simulink model "LUT_liver_pancreas_25"  (R2023b)
settings: Solver=FixedStepAuto  StartTime=0  StopTime=10.1  FixedStep=Timegap  RelTol=1e-3
model workspace (MAT data in the model file):
  T1_input = 1.34
(part 3 of 3)

== system LUT_liver_pancreas_25/If Action Subsystem6/If Action Subsystem2/If Action Subsystem9/If Action Subsystem1 ==
  In1 : Inport
  Action Port : ActionPort  ActionPortLabel=elseif( u1 >= 1.915)
  LUT 1.92RR : Lookup_n-D  NumberOfTableDimensions=1  BreakpointsForDimension1=[398.6604;505.5409;602.0864;698.3082;794.1288;889.6453;984.9397;1080.071;1175.08;1269.997;1364.843;1459.632;1554.377;1649.085;1743.765;1838.419;1933.054]  Table=[400;500;600;700;800;900;1000;1100;1200;1300;1400;1500;1600;1700;1800;1900;2000]  InternalRulePriority=Speed  RndMeth=Simplest
  Out1 : Outport
  wires:
  In1/1 -> LUT 1.92RR/1
  LUT 1.92RR/1 -> Out1/1

== system LUT_liver_pancreas_25/If Action Subsystem6/If Action Subsystem2/If Action Subsystem9/If Action Subsystem10 ==
  In1 : Inport
  Action Port : ActionPort  ActionPortLabel=if(u1 >= 1.995)
  LUT 2.00RR : Lookup_n-D  NumberOfTableDimensions=1  BreakpointsForDimension1=[398.4498;505.3086;601.8224;697.9817;793.713;889.1189;984.286;1079.277;1174.137;1268.896;1363.577;1458.198;1552.77;1647.302;1741.803;1836.277;1930.729]  Table=[400;500;600;700;800;900;1000;1100;1200;1300;1400;1500;1600;1700;1800;1900;2000]  InternalRulePriority=Speed  RndMeth=Simplest
  Out1 : Outport
  wires:
  In1/1 -> LUT 2.00RR/1
  LUT 2.00RR/1 -> Out1/1

== system LUT_liver_pancreas_25/If Action Subsystem6/If Action Subsystem2/If Action Subsystem9/If Action Subsystem11 ==
  In1 : Inport
  Action Port : ActionPort  ActionPortLabel=elseif( u1 >= 1.905)
  LUT 1.91RR : Lookup_n-D  NumberOfTableDimensions=1  BreakpointsForDimension1=[398.6878;505.5719;602.1224;698.3532;794.1862;889.7178;985.0294;1080.179;1175.209;1270.147;1365.014;1459.826;1554.593;1649.325;1744.028;1838.706;1933.365]  Table=[400;500;600;700;800;900;1000;1100;1200;1300;1400;1500;1600;1700;1800;1900;2000]  InternalRulePriority=Speed  RndMeth=Simplest
  Out1 : Outport
  wires:
  In1/1 -> LUT 1.91RR/1
  LUT 1.91RR/1 -> Out1/1

== system LUT_liver_pancreas_25/If Action Subsystem6/If Action Subsystem2/If Action Subsystem9/If Action Subsystem2 ==
  In1 : Inport
  Action Port : ActionPort  ActionPortLabel=else
  LUT 1.90RR : Lookup_n-D  NumberOfTableDimensions=1  BreakpointsForDimension1=[398.7156;505.6034;602.1591;698.3991;794.2449;889.7919;985.121;1080.29;1175.34;1270.299;1365.188;1460.023;1554.813;1649.569;1744.295;1838.998;1933.681]  Table=[400;500;600;700;800;900;1000;1100;1200;1300;1400;1500;1600;1700;1800;1900;2000]  InternalRulePriority=Speed  RndMeth=Simplest
  Out1 : Outport
  wires:
  In1/1 -> LUT 1.90RR/1
  LUT 1.90RR/1 -> Out1/1

== system LUT_liver_pancreas_25/If Action Subsystem6/If Action Subsystem2/If Action Subsystem9/If Action Subsystem3 ==
  In1 : Inport
  Action Port : ActionPort  ActionPortLabel=elseif( u1 >= 1.925)
  LUT 1.93RR : Lookup_n-D  NumberOfTableDimensions=1  BreakpointsForDimension1=[398.6331;505.5103;602.0511;698.2642;794.0727;889.5743;984.8519;1079.965;1174.954;1269.851;1364.675;1459.442;1554.164;1648.85;1743.505;1838.137;1932.747]  Table=[400;500;600;700;800;900;1000;1100;1200;1300;1400;1500;1600;1700;1800;1900;2000]  InternalRulePriority=Speed  RndMeth=Simplest
  Out1 : Outport
  wires:
  In1/1 -> LUT 1.93RR/1
  LUT 1.93RR/1 -> Out1/1

== system LUT_liver_pancreas_25/If Action Subsystem6/If Action Subsystem2/If Action Subsystem9/If Action Subsystem4 ==
  In1 : Inport
  Action Port : ActionPort  ActionPortLabel=elseif( u1 >= 1.935)
  LUT 1.94RR : Lookup_n-D  NumberOfTableDimensions=1  BreakpointsForDimension1=[398.6062;505.4802;602.0165;698.2211;794.0178;889.5049;984.7658;1079.86;1174.831;1269.706;1364.509;1459.255;1553.955;1648.618;1743.25;1837.858;1932.446]  Table=[400;500;600;700;800;900;1000;1100;1200;1300;1400;1500;1600;1700;1800;1900;2000]  InternalRulePriority=Speed  RndMeth=Simplest
  Out1 : Outport
  wires:
  In1/1 -> LUT 1.94RR/1
  LUT 1.94RR/1 -> Out1/1

== system LUT_liver_pancreas_25/If Action Subsystem6/If Action Subsystem2/If Action Subsystem9/If Action Subsystem5 ==
  In1 : Inport
  Action Port : ActionPort  ActionPortLabel=elseif( u1 >= 1.955)
  LUT 1.96RR : Lookup_n-D  NumberOfTableDimensions=1  BreakpointsForDimension1=[398.5531;505.4213;601.9493;698.1378;793.9116;889.3705;984.5991;1079.658;1174.59;1269.426;1364.187;1458.89;1553.546;1648.165;1742.752;1837.315;1931.856]  Table=[400;500;600;700;800;900;1000;1100;1200;1300;1400;1500;1600;1700;1800;1900;2000]  InternalRulePriority=Speed  RndMeth=Simplest
  Out1 : Outport
  wires:
  In1/1 -> LUT 1.96RR/1
  LUT 1.96RR/1 -> Out1/1

== system LUT_liver_pancreas_25/If Action Subsystem6/If Action Subsystem2/If Action Subsystem9/If Action Subsystem6 ==
  In1 : Inport
  Action Port : ActionPort  ActionPortLabel=elseif( u1 >= 1.945)
  LUT 1.95RR : Lookup_n-D  NumberOfTableDimensions=1  BreakpointsForDimension1=[398.5795;505.4506;601.9826;698.179;793.9641;889.437;984.6816;1079.758;1174.709;1269.565;1364.347;1459.071;1553.749;1648.389;1742.999;1837.585;1932.149]  Table=[400;500;600;700;800;900;1000;1100;1200;1300;1400;1500;1600;1700;1800;1900;2000]  InternalRulePriority=Speed  RndMeth=Simplest
  Out1 : Outport
  wires:
  In1/1 -> LUT 1.95RR/1
  LUT 1.95RR/1 -> Out1/1

== system LUT_liver_pancreas_25/If Action Subsystem6/If Action Subsystem2/If Action Subsystem9/If Action Subsystem7 ==
  In1 : Inport
  Action Port : ActionPort  ActionPortLabel=elseif( u1 >= 1.965)
  LUT 1.97RR : Lookup_n-D  NumberOfTableDimensions=1  BreakpointsForDimension1=[398.5269;505.3925;601.9166;698.0975;793.8603;889.3055;984.5183;1079.56;1174.473;1269.29;1364.031;1458.712;1553.347;1647.944;1742.509;1837.049;1931.568]  Table=[400;500;600;700;800;900;1000;1100;1200;1300;1400;1500;1600;1700;1800;1900;2000]  InternalRulePriority=Speed  RndMeth=Simplest
  Out1 : Outport
  wires:
  In1/1 -> LUT 1.97RR/1
  LUT 1.97RR/1 -> Out1/1

== system LUT_liver_pancreas_25/If Action Subsystem6/If Action Subsystem2/If Action Subsystem9/If Action Subsystem8 ==
  In1 : Inport
  Action Port : ActionPort  ActionPortLabel=elseif( u1 >= 1.975)
  LUT 1.98RR : Lookup_n-D  NumberOfTableDimensions=1  BreakpointsForDimension1=[398.501;505.3641;601.8846;698.058;793.8101;889.2419;984.4392;1079.464;1174.359;1269.156;1363.877;1458.538;1553.151;1647.726;1742.27;1836.788;1931.284]  Table=[400;500;600;700;800;900;1000;1100;1200;1300;1400;1500;1600;1700;1800;1900;2000]  InternalRulePriority=Speed  RndMeth=Simplest
  Out1 : Outport
  wires:
  In1/1 -> LUT 1.98RR/1
  LUT 1.98RR/1 -> Out1/1

== system LUT_liver_pancreas_25/If Action Subsystem6/If Action Subsystem2/If Action Subsystem9/If Action Subsystem9 ==
  In1 : Inport
  Action Port : ActionPort  ActionPortLabel=elseif(u1 >= 1.985)
  LUT 1.99RR : Lookup_n-D  NumberOfTableDimensions=1  BreakpointsForDimension1=[398.4753;505.3361;601.8532;698.0194;793.761;889.1797;984.3618;1079.369;1174.247;1269.025;1363.726;1458.366;1552.959;1647.513;1742.035;1836.53;1931.004]  Table=[400;500;600;700;800;900;1000;1100;1200;1300;1400;1500;1600;1700;1800;1900;2000]  InternalRulePriority=Speed  RndMeth=Simplest
  Out1 : Outport
  wires:
  In1/1 -> LUT 1.99RR/1
  LUT 1.99RR/1 -> Out1/1

== system LUT_liver_pancreas_25/If Action Subsystem6/If Action Subsystem3/If Action Subsystem5/If Action Subsystem1 ==
  In1 : Inport
  Action Port : ActionPort  ActionPortLabel=elseif( u1 >= 0.615)
  LUT 0.62RR : Lookup_n-D  NumberOfTableDimensions=1  BreakpointsForDimension1=[413.0526;530.6767;636.9684;743.5036;850.0094;956.4958;1063.005;1169.582;1276.273;1383.115;1490.11;1597.539;1705.059;1812.916;1921.116;2029.689;2138.661]  Table=[400;500;600;700;800;900;1000;1100;1200;1300;1400;1500;1600;1700;1800;1900;2000]  InternalRulePriority=Speed  RndMeth=Simplest
  Out1 : Outport
  wires:
  In1/1 -> LUT 0.62RR/1
  LUT 0.62RR/1 -> Out1/1

== system LUT_liver_pancreas_25/If Action Subsystem6/If Action Subsystem3/If Action Subsystem5/If Action Subsystem10 ==
  In1 : Inport
  Action Port : ActionPort  ActionPortLabel=elseif( u1 >= 0.605)
  LUT 0.61RR : Lookup_n-D  NumberOfTableDimensions=1  BreakpointsForDimension1=[413.6063;531.8654;638.6532;745.6537;852.6076;959.5359;1066.49;1173.523;1280.687;1388.021;1504.644;1603.565;1711.69;1820.197;1929.1;2038.429;2148.217]  Table=[400;500;600;700;800;900;1000;1100;1200;1300;1400;1500;1600;1700;1800;1900;2000]  InternalRulePriority=Speed  RndMeth=Simplest
  Out1 : Outport
  wires:
  In1/1 -> LUT 0.61RR/1
  LUT 0.61RR/1 -> Out1/1

== system LUT_liver_pancreas_25/If Action Subsystem6/If Action Subsystem3/If Action Subsystem5/If Action Subsystem2 ==
  In1 : Inport
  Action Port : ActionPort  ActionPortLabel=else
  LUT 0.6RR : Lookup_n-D  NumberOfTableDimensions=1  BreakpointsForDimension1=[414.1881;533.143;640.4713;747.9759;855.4138;962.8193;1070.254;1177.781;1285.457;1393.325;1505.695;1610.101;1718.894;1828.12;1937.801;2047.972;2158.67]  Table=[400;500;600;700;800;900;1000;1100;1200;1300;1400;1500;1600;1700;1800;1900;2000]  InternalRulePriority=Speed  RndMeth=Simplest
  Out1 : Outport
  wires:
  In1/1 -> LUT 0.6RR/1
  LUT 0.6RR/1 -> Out1/1

== system LUT_liver_pancreas_25/If Action Subsystem6/If Action Subsystem3/If Action Subsystem5/If Action Subsystem3 ==
  In1 : Inport
  Action Port : ActionPort  ActionPortLabel=elseif( u1 >= 0.625)
  LUT 0.63RR : Lookup_n-D  NumberOfTableDimensions=1  BreakpointsForDimension1=[412.5257;529.5692;635.4041;741.5087;847.5987;953.6745;1059.77;1165.926;1272.179;1378.566;1485.105;1591.969;1698.936;1806.202;1913.768;2021.658;2129.896]  Table=[400;500;600;700;800;900;1000;1100;1200;1300;1400;1500;1600;1700;1800;1900;2000]  InternalRulePriority=Speed  RndMeth=Simplest
  Out1 : Outport
  wires:
  In1/1 -> LUT 0.63RR/1
  LUT 0.63RR/1 -> Out1/1

== system LUT_liver_pancreas_25/If Action Subsystem6/If Action Subsystem3/If Action Subsystem5/If Action Subsystem4 ==
  In1 : Inport
  Action Port : ActionPort  ActionPortLabel=elseif( u1 >= 0.635)
  LUT 0.64RR : Lookup_n-D  NumberOfTableDimensions=1  BreakpointsForDimension1=[412.0245;528.5358;633.9491;739.6539;845.3569;951.0501;1056.761;1162.524;1268.371;1374.335;1480.441;1586.807;1693.265;1799.994;1906.983;2014.254;2121.83]  Table=[400;500;600;700;800;900;1000;1100;1200;1300;1400;1500;1600;1700;1800;1900;2000]  InternalRulePriority=Speed  RndMeth=Simplest
  Out1 : Outport
  wires:
  In1/1 -> LUT 0.64RR/1
  LUT 0.64RR/1 -> Out1/1

== system LUT_liver_pancreas_25/If Action Subsystem6/If Action Subsystem3/If Action Subsystem5/If Action Subsystem5 ==
  In1 : Inport
  Action Port : ActionPort  ActionPortLabel=elseif( u1 >= 0.655)
  LUT 0.66RR : Lookup_n-D  NumberOfTableDimensions=1  BreakpointsForDimension1=[411.0948;526.6663;631.3276;736.3133;841.3167;946.3174;1051.332;1156.386;1261.503;1366.708;1472.025;1580.011;1683.093;1788.878;1894.86;2001.057;2107.487]  Table=[400;500;600;700;800;900;1000;1100;1200;1300;1400;1500;1600;1700;1800;1900;2000]  InternalRulePriority=Speed  RndMeth=Simplest
  Out1 : Outport
  wires:
  In1/1 -> LUT 0.66RR/1
  LUT 0.66RR/1 -> Out1/1

== system LUT_liver_pancreas_25/If Action Subsystem6/If Action Subsystem3/If Action Subsystem5/If Action Subsystem6 ==
  In1 : Inport
  Action Port : ActionPort  ActionPortLabel=elseif( u1 >= 0.645)
  LUT 0.65RR : Lookup_n-D  NumberOfTableDimensions=1  BreakpointsForDimension1=[411.548;527.57;632.5933;737.9261;843.2677;948.6034;1053.955;1159.351;1264.821;1370.392;1476.091;1582.028;1687.998;1794.235;1900.698;2007.408;2114.383]  Table=[400;500;600;700;800;900;1000;1100;1200;1300;1400;1500;1600;1700;1800;1900;2000]  InternalRulePriority=Speed  RndMeth=Simplest
  Out1 : Outport
  wires:
  In1/1 -> LUT 0.65RR/1
  LUT 0.65RR/1 -> Out1/1

== system LUT_liver_pancreas_25/If Action Subsystem6/If Action Subsystem3/If Action Subsystem5/If Action Subsystem7 ==
  In1 : Inport
  Action Port : ActionPort  ActionPortLabel=elseif( u1 >= 0.665)
  LUT 0.67RR : Lookup_n-D  NumberOfTableDimensions=1  BreakpointsForDimension1=[410.6639;525.8193;630.1439;734.805;839.491;944.177;1048.876;1153.607;1258.394;1363.258;1468.219;1581.997;1678.512;1783.881;1889.421;1995.149;2101.08]  Table=[400;500;600;700;800;900;1000;1100;1200;1300;1400;1500;1600;1700;1800;1900;2000]  InternalRulePriority=Speed  RndMeth=Simplest
  Out1 : Outport
  wires:
  In1/1 -> LUT 0.67RR/1
  LUT 0.67RR/1 -> Out1/1

== system LUT_liver_pancreas_25/If Action Subsystem6/If Action Subsystem3/If Action Subsystem5/If Action Subsystem8 ==
  In1 : Inport
  Action Port : ActionPort  ActionPortLabel=elseif(u1 >= 0.675)
  LUT 0.68RR : Lookup_n-D  NumberOfTableDimensions=1  BreakpointsForDimension1=[410.2541;525.0244;629.0351;733.3917;837.7791;942.1686;1046.569;1150.998;1255.475;1360.018;1464.646;1569.375;1674.224;1779.207;1884.339;1989.636;2095.11]  Table=[400;500;600;700;800;900;1000;1100;1200;1300;1400;1500;1600;1700;1800;1900;2000]  InternalRulePriority=Speed  RndMeth=Simplest
  Out1 : Outport
  wires:
  In1/1 -> LUT 0.68RR/1
  LUT 0.68RR/1 -> Out1/1

== system LUT_liver_pancreas_25/If Action Subsystem6/If Action Subsystem3/If Action Subsystem5/If Action Subsystem9 ==
  In1 : Inport
  Action Port : ActionPort  ActionPortLabel=if(u1 >= 0.685)
  LUT 0.69RR : Lookup_n-D  NumberOfTableDimensions=1  BreakpointsForDimension1=[409.7732;524.2774;627.9946;732.0649;836.1708;940.2803;1044.4;1148.543;1252.728;1356.97;1461.285;1565.687;1670.201;1774.824;1879.579;1984.478;2089.532]  Table=[400;500;600;700;800;900;1000;1100;1200;1300;1400;1500;1600;1700;1800;1900;2000]  InternalRulePriority=Speed  RndMeth=Simplest
  Out1 : Outport
  wires:
  In1/1 -> LUT 0.69RR/1
  LUT 0.69RR/1 -> Out1/1

== system LUT_liver_pancreas_25/If Action Subsystem6/If Action Subsystem3/If Action Subsystem6/If Action Subsystem1 ==
  In1 : Inport
  Action Port : ActionPort  ActionPortLabel=elseif( u1 >= 0.515)
  LUT 0.52RR : Lookup_n-D  NumberOfTableDimensions=1  BreakpointsForDimension1=[419.925;547.8462;661.9676;775.6675;888.9962;1002.208;1115.536;1229.174;1343.225;1459.982;1574.478;1691.12;1808.984;1928.148;2048.731;2170.858;2294.661]  Table=[400;500;600;700;800;900;1000;1100;1200;1300;1400;1500;1600;1700;1800;1900;2000]  InternalRulePriority=Speed  RndMeth=Simplest
  Out1 : Outport
  wires:
  In1/1 -> LUT 0.52RR/1
  LUT 0.52RR/1 -> Out1/1

== system LUT_liver_pancreas_25/If Action Subsystem6/If Action Subsystem3/If Action Subsystem6/If Action Subsystem10 ==
  In1 : Inport
  Action Port : ActionPort  ActionPortLabel=elseif( u1 >= 0.505)
  LUT 0.51RR : Lookup_n-D  NumberOfTableDimensions=1  BreakpointsForDimension1=[420.7723;550.4608;665.9025;780.7905;895.2445;1009.57;1124.038;1238.87;1354.163;1471.848;1588.432;1706.804;1826.569;1947.837;2070.753;2195.464;2322.135]  Table=[400;500;600;700;800;900;1000;1100;1200;1300;1400;1500;1600;1700;1800;1900;2000]  InternalRulePriority=Speed  RndMeth=Simplest
  Out1 : Outport
  wires:
  In1/1 -> LUT 0.51RR/1
  LUT 0.51RR/1 -> Out1/1

== system LUT_liver_pancreas_25/If Action Subsystem6/If Action Subsystem3/If Action Subsystem6/If Action Subsystem2 ==
  In1 : Inport
  Action Port : ActionPort  ActionPortLabel=else
  LUT 0.50RR : Lookup_n-D  NumberOfTableDimensions=1  BreakpointsForDimension1=[421.6409;553.3122;670.2323;786.4478;902.1595;1017.731;1133.48;1249.661;1366.356;1485.421;1604.038;1724.383;1846.324;1970.008;2095.608;2223.304;2353.3]  Table=[400;500;600;700;800;900;1000;1100;1200;1300;1400;1500;1600;1700;1800;1900;2000]  InternalRulePriority=Speed  RndMeth=Simplest
  Out1 : Outport
  wires:
  In1/1 -> LUT 0.50RR/1
  LUT 0.50RR/1 -> Out1/1

== system LUT_liver_pancreas_25/If Action Subsystem6/If Action Subsystem3/If Action Subsystem6/If Action Subsystem3 ==
  In1 : Inport
  Action Port : ActionPort  ActionPortLabel=elseif( u1 >= 0.525)
  LUT 0.53RR : Lookup_n-D  NumberOfTableDimensions=1  BreakpointsForDimension1=[419.1032;545.4456;658.3845;771.0177;883.336;995.5501;1107.859;1220.432;1333.374;1450.068;1561.96;1677.078;1793.276;1910.599;2029.148;2149.026;2270.345]  Table=[400;500;600;700;800;900;1000;1100;1200;1300;1400;1500;1600;1700;1800;1900;2000]  InternalRulePriority=Speed  RndMeth=Simplest
  Out1 : Outport
  wires:
  In1/1 -> LUT 0.53RR/1
  LUT 0.53RR/1 -> Out1/1

== system LUT_liver_pancreas_25/If Action Subsystem6/If Action Subsystem3/If Action Subsystem6/If Action Subsystem4 ==
  In1 : Inport
  Action Port : ActionPort  ActionPortLabel=elseif( u1 >= 0.535)
  LUT 0.54RR : Lookup_n-D  NumberOfTableDimensions=1  BreakpointsForDimension1=[418.3095;543.2384;655.1154;766.7878;878.1954;989.5111;1100.905;1212.525;1324.473;1442.464;1550.696;1664.462;1779.194;1894.902;2011.67;2129.586;2248.743]  Table=[400;500;600;700;800;900;1000;1100;1200;1300;1400;1500;1600;1700;1800;1900;2000]  InternalRulePriority=Speed  RndMeth=Simplest
  Out1 : Outport
  wires:
  In1/1 -> LUT 0.54RR/1
  LUT 0.54RR/1 -> Out1/1

== system LUT_liver_pancreas_25/If Action Subsystem6/If Action Subsystem3/If Action Subsystem6/If Action Subsystem5 ==
  In1 : Inport
  Action Port : ActionPort  ActionPortLabel=elseif( u1 >= 0.555)
  LUT 0.56RR : Lookup_n-D  NumberOfTableDimensions=1  BreakpointsForDimension1=[416.8124;538.8983;649.3892;759.4066;869.2429;979.0103;1088.832;1198.821;1309.064;1419.513;1531.335;1642.805;1755.093;1868.119;1981.942;2096.624;2212.235]  Table=[400;500;600;700;800;900;1000;1100;1200;1300;1400;1500;1600;1700;1800;1900;2000]  InternalRulePriority=Speed  RndMeth=Simplest
  Out1 : Outport
  wires:
  In1/1 -> LUT 0.56RR/1
  LUT 0.56RR/1 -> Out1/1

== system LUT_liver_pancreas_25/If Action Subsystem6/If Action Subsystem3/If Action Subsystem6/If Action Subsystem6 ==
  In1 : Inport
  Action Port : ActionPort  ActionPortLabel=elseif( u1 >= 0.545)
  LUT 0.55RR : Lookup_n-D  NumberOfTableDimensions=1  BreakpointsForDimension1=[417.5456;541.1396;652.1268;762.9311;873.515;984.0188;1094.588;1205.35;1316.403;1436.98;1540.531;1653.091;1766.527;1880.812;1996.014;2112.21;2229.478]  Table=[400;500;600;700;800;900;1000;1100;1200;1300;1400;1500;1600;1700;1800;1900;2000]  InternalRulePriority=Speed  RndMeth=Simplest
  Out1 : Outport
  wires:
  In1/1 -> LUT 0.55RR/1
  LUT 0.55RR/1 -> Out1/1

== system LUT_liver_pancreas_25/If Action Subsystem6/If Action Subsystem3/If Action Subsystem6/If Action Subsystem7 ==
  In1 : Inport
  Action Port : ActionPort  ActionPortLabel=elseif( u1 >= 0.565)
  LUT 0.57RR : Lookup_n-D  NumberOfTableDimensions=1  BreakpointsForDimension1=[416.1104;536.8576;646.8766;756.1785;865.3339;974.4308;1083.574;1192.86;1302.37;1412.111;1523.01;1633.472;1744.736;1856.646;1969.247;2082.593;2196.744]  Table=[400;500;600;700;800;900;1000;1100;1200;1300;1400;1500;1600;1700;1800;1900;2000]  InternalRulePriority=Speed  RndMeth=Simplest
  Out1 : Outport
  wires:
  In1/1 -> LUT 0.57RR/1
  LUT 0.57RR/1 -> Out1/1

== system LUT_liver_pancreas_25/If Action Subsystem6/If Action Subsystem3/If Action Subsystem6/If Action Subsystem8 ==
  In1 : Inport
  Action Port : ActionPort  ActionPortLabel=elseif(u1 >= 0.575)
  LUT 0.58RR : Lookup_n-D  NumberOfTableDimensions=1  BreakpointsForDimension1=[415.4393;536.0008;644.566;753.2153;861.7484;970.2327;1078.756;1187.403;1296.246;1405.316;1515.517;1624.974;1735.325;1846.24;1957.755;2069.918;2182.779]  Table=[400;500;600;700;800;900;1000;1100;1200;1300;1400;1500;1600;1700;1800;1900;2000]  InternalRulePriority=Speed  RndMeth=Simplest
  Out1 : Outport
  wires:
  In1/1 -> LUT 0.58RR/1
  LUT 0.58RR/1 -> Out1/1

== system LUT_liver_pancreas_25/If Action Subsystem6/If Action Subsystem3/If Action Subsystem6/If Action Subsystem9 ==
  In1 : Inport
  Action Port : ActionPort  ActionPortLabel=if(u1 >= 0.585)
  LUT 0.59RR : Lookup_n-D  NumberOfTableDimensions=1  BreakpointsForDimension1=[414.7988;534.5182;642.4369;750.4892;858.4519;966.3743;1074.331;1182.393;1290.627;1399.073;1509.163;1617.212;1726.743;1836.769;1947.315;2058.426;2170.143]  Table=[400;500;600;700;800;900;1000;1100;1200;1300;1400;1500;1600;1700;1800;1900;2000]  InternalRulePriority=Speed  RndMeth=Simplest
  Out1 : Outport
  wires:
  In1/1 -> LUT 0.59RR/1
  LUT 0.59RR/1 -> Out1/1

== system LUT_liver_pancreas_25/If Action Subsystem6/If Action Subsystem3/If Action Subsystem7/If Action Subsystem1 ==
  In1 : Inport
  Action Port : ActionPort  ActionPortLabel=elseif( u1 >= 0.715)
  LUT 0.72RR : Lookup_n-D  NumberOfTableDimensions=1  BreakpointsForDimension1=[408.8044;522.2865;625.2275;728.5323;831.8808;935.2351;1038.595;1141.97;1245.37;1348.806;1452.289;1555.826;1661.357;1763.155;1866.924;1970.794;2074.77]  Table=[400;500;600;700;800;900;1000;1100;1200;1300;1400;1500;1600;1700;1800;1900;2000]  InternalRulePriority=Speed  RndMeth=Simplest
  Out1 : Outport
  wires:
  In1/1 -> LUT 0.72RR/1
  LUT 0.72RR/1 -> Out1/1

== system LUT_liver_pancreas_25/If Action Subsystem6/If Action Subsystem3/If Action Subsystem7/If Action Subsystem10 ==
  In1 : Inport
  Action Port : ActionPort  ActionPortLabel=elseif( u1 >= 0.705)
  LUT 0.71RR : Lookup_n-D  NumberOfTableDimensions=1  BreakpointsForDimension1=[409.1404;522.9118;626.0958;729.6417;833.2294;936.8226;1040.423;1144.041;1247.688;1351.378;1455.123;1558.931;1662.9;1766.82;1870.898;1975.087;2079.395]  Table=[400;500;600;700;800;900;1000;1100;1200;1300;1400;1500;1600;1700;1800;1900;2000]  InternalRulePriority=Speed  RndMeth=Simplest
  Out1 : Outport
  wires:
  In1/1 -> LUT 0.71RR/1
  LUT 0.71RR/1 -> Out1/1

== system LUT_liver_pancreas_25/If Action Subsystem6/If Action Subsystem3/If Action Subsystem7/If Action Subsystem2 ==
  In1 : Inport
  Action Port : ActionPort  ActionPortLabel=else
  LUT 0.70RR : Lookup_n-D  NumberOfTableDimensions=1  BreakpointsForDimension1=[409.5212;523.5744;627.0166;730.8172;834.657;938.5015;1042.354;1146.228;1250.137;1354.095;1458.116;1562.212;1666.423;1770.703;1875.108;1979.638;2084.306]  Table=[400;500;600;700;800;900;1000;1100;1200;1300;1400;1500;1600;1700;1800;1900;2000]  InternalRulePriority=Speed  RndMeth=Simplest
  Out1 : Outport
  wires:
  In1/1 -> LUT 0.70RR/1
  LUT 0.70RR/1 -> Out1/1

== system LUT_liver_pancreas_25/If Action Subsystem6/If Action Subsystem3/If Action Subsystem7/If Action Subsystem3 ==
  In1 : Inport
  Action Port : ActionPort  ActionPortLabel=elseif( u1 >= 0.725)
  LUT 0.73RR : Lookup_n-D  NumberOfTableDimensions=1  BreakpointsForDimension1=[408.4842;521.6957;624.4073;727.4836;830.6046;933.7314;1036.863;1140.006;1243.171;1346.366;1449.601;1552.882;1665.038;1759.687;1863.165;1966.738;2070.403]  Table=[400;500;600;700;800;900;1000;1100;1200;1300;1400;1500;1600;1700;1800;1900;2000]  InternalRulePriority=Speed  RndMeth=Simplest
  Out1 : Outport
  wires:
  In1/1 -> LUT 0.73RR/1
  LUT 0.73RR/1 -> Out1/1

== system LUT_liver_pancreas_25/If Action Subsystem6/If Action Subsystem3/If Action Subsystem7/If Action Subsystem4 ==
  In1 : Inport
  Action Port : ActionPort  ActionPortLabel=elseif( u1 >= 0.735)
  LUT 0.74RR : Lookup_n-D  NumberOfTableDimensions=1  BreakpointsForDimension1=[408.1791;521.1367;623.6316;726.4907;829.3949;932.3046;1035.218;1138.14;1241.08;1344.046;1447.047;1550.086;1653.132;1756.403;1859.603;1962.895;2066.27]  Table=[400;500;600;700;800;900;1000;1100;1200;1300;1400;1500;1600;1700;1800;1900;2000]  InternalRulePriority=Speed  RndMeth=Simplest
  Out1 : Outport
  wires:
  In1/1 -> LUT 0.74RR/1
  LUT 0.74RR/1 -> Out1/1

== system LUT_liver_pancreas_25/If Action Subsystem6/If Action Subsystem3/If Action Subsystem7/If Action Subsystem5 ==
  In1 : Inport
  Action Port : ActionPort  ActionPortLabel=elseif( u1 >= 0.755)
  LUT 0.76RR : Lookup_n-D  NumberOfTableDimensions=1  BreakpointsForDimension1=[407.6106;520.1046;622.1995;724.6547;827.1542;929.6577;1032.162;1134.671;1237.192;1339.732;1442.295;1544.886;1647.491;1750.366;1852.999;1955.777;2058.623]  Table=[400;500;600;700;800;900;1000;1100;1200;1300;1400;1500;1600;1700;1800;1900;2000]  InternalRulePriority=Speed  RndMeth=Simplest
  Out1 : Outport
  wires:
  In1/1 -> LUT 0.76RR/1
  LUT 0.76RR/1 -> Out1/1

== system LUT_liver_pancreas_25/If Action Subsystem6/If Action Subsystem3/If Action Subsystem7/If Action Subsystem6 ==
  In1 : Inport
  Action Port : ActionPort  ActionPortLabel=elseif( u1 >= 0.745)
  LUT 0.75RR : Lookup_n-D  NumberOfTableDimensions=1  BreakpointsForDimension1=[407.8882;520.607;622.8967;725.549;828.2464;930.9486;1033.653;1136.364;1239.09;1341.838;1444.614;1547.424;1650.246;1753.294;1856.219;1959.247;2062.35]  Table=[400;500;600;700;800;900;1000;1100;1200;1300;1400;1500;1600;1700;1800;1900;2000]  InternalRulePriority=Speed  RndMeth=Simplest
  Out1 : Outport
  wires:
  In1/1 -> LUT 0.75RR/1
  LUT 0.75RR/1 -> Out1/1

== system LUT_liver_pancreas_25/If Action Subsystem6/If Action Subsystem3/If Action Subsystem7/If Action Subsystem7 ==
  In1 : Inport
  Action Port : ActionPort  ActionPortLabel=elseif( u1 >= 0.765)
  LUT 0.77RR : Lookup_n-D  NumberOfTableDimensions=1  BreakpointsForDimension1=[407.3457;519.4328;621.5371;723.8041;826.1141;928.4272;1030.74;1133.055;1235.38;1337.719;1440.079;1542.462;1644.858;1747.712;1849.931;1952.47;2055.074]  Table=[400;500;600;700;800;900;1000;1100;1200;1300;1400;1500;1600;1700;1800;1900;2000]  InternalRulePriority=Speed  RndMeth=Simplest
  Out1 : Outport
  wires:
  In1/1 -> LUT 0.77RR/1
  LUT 0.77RR/1 -> Out1/1

== system LUT_liver_pancreas_25/If Action Subsystem6/If Action Subsystem3/If Action Subsystem7/If Action Subsystem8 ==
  In1 : Inport
  Action Port : ActionPort  ActionPortLabel=elseif(u1 >= 0.775)
  LUT 0.78RR : Lookup_n-D  NumberOfTableDimensions=1  BreakpointsForDimension1=[407.0925;519.1024;620.9069;722.9938;825.1221;927.2523;1029.38;1131.51;1233.646;1335.794;1437.959;1540.144;1642.339;1746.985;1847.004;1949.313;2051.688]  Table=[400;500;600;700;800;900;1000;1100;1200;1300;1400;1500;1600;1700;1800;1900;2000]  InternalRulePriority=Speed  RndMeth=Simplest
  Out1 : Outport
  wires:
  In1/1 -> LUT 0.78RR/1
  LUT 0.78RR/1 -> Out1/1

== system LUT_liver_pancreas_25/If Action Subsystem6/If Action Subsystem3/If Action Subsystem7/If Action Subsystem9 ==
  In1 : Inport
  Action Port : ActionPort  ActionPortLabel=if(u1 >= 0.785)
  LUT 0.79RR : Lookup_n-D  NumberOfTableDimensions=1  BreakpointsForDimension1=[406.8506;518.7905;620.3067;722.221;824.1748;926.1291;1028.08;1130.03;1231.986;1333.95;1435.928;1537.922;1639.926;1741.712;1844.209;1946.294;2048.451]  Table=[400;500;600;700;800;900;1000;1100;1200;1300;1400;1500;1600;1700;1800;1900;2000]  InternalRulePriority=Speed  RndMeth=Simplest
  Out1 : Outport
  wires:
  In1/1 -> LUT 0.79RR/1
  LUT 0.79RR/1 -> Out1/1

== system LUT_liver_pancreas_25/If Action Subsystem6/If Action Subsystem3/If Action Subsystem8/If Action Subsystem1 ==
  In1 : Inport
  Action Port : ActionPort  ActionPortLabel=elseif( u1 >= 0.815)
  LUT 0.82RR : Lookup_n-D  NumberOfTableDimensions=1  BreakpointsForDimension1=[406.1853;517.5611;618.6645;720.1013;821.5701;923.0343;1024.491;1125.942;1227.393;1328.846;1430.306;1531.774;1633.247;1734.683;1836.627;1937.969;2039.525]  Table=[400;500;600;700;800;900;1000;1100;1200;1300;1400;1500;1600;1700;1800;1900;2000]  InternalRulePriority=Speed  RndMeth=Simplest
  Out1 : Outport
  wires:
  In1/1 -> LUT 0.82RR/1
  LUT 0.82RR/1 -> Out1/1

== system LUT_liver_pancreas_25/If Action Subsystem6/If Action Subsystem3/If Action Subsystem8/If Action Subsystem10 ==
  In1 : Inport
  Action Port : ActionPort  ActionPortLabel=elseif( u1 >= 0.805)
  LUT 0.81RR : Lookup_n-D  NumberOfTableDimensions=1  BreakpointsForDimension1=[406.3976;517.9366;619.1873;720.7771;822.4016;924.0233;1025.639;1127.251;1228.863;1330.481;1432.107;1533.744;1635.387;1736.972;1839.006;1940.63;2042.379]  Table=[400;500;600;700;800;900;1000;1100;1200;1300;1400;1500;1600;1700;1800;1900;2000]  InternalRulePriority=Speed  RndMeth=Simplest
  Out1 : Outport
  wires:
  In1/1 -> LUT 0.81RR/1
  LUT 0.81RR/1 -> Out1/1

== system LUT_liver_pancreas_25/If Action Subsystem6/If Action Subsystem3/If Action Subsystem8/If Action Subsystem2 ==
  In1 : Inport
  Action Port : ActionPort  ActionPortLabel=else
  LUT 0.80RR : Lookup_n-D  NumberOfTableDimensions=1  BreakpointsForDimension1=[406.6191;518.4954;619.7341;721.4829;823.2689;925.0539;1026.834;1128.612;1230.393;1332.181;1433.979;1535.791;1637.611;1739.331;1841.542;1943.403;2045.351]  Table=[400;500;600;700;800;900;1000;1100;1200;1300;1400;1500;1600;1700;1800;1900;2000]  InternalRulePriority=Speed  RndMeth=Simplest
  Out1 : Outport
  wires:
  In1/1 -> LUT 0.80RR/1
  LUT 0.80RR/1 -> Out1/1

== system LUT_liver_pancreas_25/If Action Subsystem6/If Action Subsystem3/If Action Subsystem8/If Action Subsystem3 ==
  In1 : Inport
  Action Port : ActionPort  ActionPortLabel=elseif( u1 >= 0.825)
  LUT 0.83RR : Lookup_n-D  NumberOfTableDimensions=1  BreakpointsForDimension1=[405.9819;517.202;618.1641;719.4536;820.7721;922.0842;1023.387;1124.683;1225.977;1327.272;1428.572;1529.877;1631.187;1732.47;1834.573;1935.412;2036.78]  Table=[400;500;600;700;800;900;1000;1100;1200;1300;1400;1500;1600;1700;1800;1900;2000]  InternalRulePriority=Speed  RndMeth=Simplest
  Out1 : Outport
  wires:
  In1/1 -> LUT 0.83RR/1
  LUT 0.83RR/1 -> Out1/1

== system LUT_liver_pancreas_25/If Action Subsystem6/If Action Subsystem3/If Action Subsystem8/If Action Subsystem4 ==
  In1 : Inport
  Action Port : ActionPort  ActionPortLabel=elseif( u1 >= 0.835)
  LUT 0.84RR : Lookup_n-D  NumberOfTableDimensions=1  BreakpointsForDimension1=[405.7867;516.8582;617.6845;718.8321;820.0055;921.1704;1022.324;1123.471;1224.613;1325.755;1426.9;1528.049;1629.2;1730.332;1834.661;1932.955;2034.138]  Table=[400;500;600;700;800;900;1000;1100;1200;1300;1400;1500;1600;1700;1800;1900;2000]  InternalRulePriority=Speed  RndMeth=Simplest
  Out1 : Outport
  wires:
  In1/1 -> LUT 0.84RR/1
  LUT 0.84RR/1 -> Out1/1

== system LUT_liver_pancreas_25/If Action Subsystem6/If Action Subsystem3/If Action Subsystem8/If Action Subsystem5 ==
  In1 : Inport
  Action Port : ActionPort  ActionPortLabel=elseif( u1 >= 0.855)
  LUT 0.86RR : Lookup_n-D  NumberOfTableDimensions=1  BreakpointsForDimension1=[405.4192;516.2125;616.7827;717.661;818.5583;919.443;1020.313;1121.173;1222.027;1322.877;1423.727;1524.579;1625.43;1726.269;1826.921;1928.331;2029.135]  Table=[400;500;600;700;800;900;1000;1100;1200;1300;1400;1500;1600;1700;1800;1900;2000]  InternalRulePriority=Speed  RndMeth=Simplest
  Out1 : Outport
  wires:
  In1/1 -> LUT 0.86RR/1
  LUT 0.86RR/1 -> Out1/1

== system LUT_liver_pancreas_25/If Action Subsystem6/If Action Subsystem3/If Action Subsystem8/If Action Subsystem6 ==
  In1 : Inport
  Action Port : ActionPort  ActionPortLabel=elseif( u1 >= 0.845)
  LUT 0.85RR : Lookup_n-D  NumberOfTableDimensions=1  BreakpointsForDimension1=[405.5993;516.5287;617.2245;718.2351;819.2682;920.2907;1021.301;1122.302;1223.297;1324.291;1425.286;1526.284;1627.283;1728.266;1828.853;1930.594;2031.591]  Table=[400;500;600;700;800;900;1000;1100;1200;1300;1400;1500;1600;1700;1800;1900;2000]  InternalRulePriority=Speed  RndMeth=Simplest
  Out1 : Outport
  wires:
  In1/1 -> LUT 0.85RR/1
  LUT 0.85RR/1 -> Out1/1

== system LUT_liver_pancreas_25/If Action Subsystem6/If Action Subsystem3/If Action Subsystem8/If Action Subsystem7 ==
  In1 : Inport
  Action Port : ActionPort  ActionPortLabel=elseif( u1 >= 0.865)
  LUT 0.87RR : Lookup_n-D  NumberOfTableDimensions=1  BreakpointsForDimension1=[405.2461;515.909;616.3581;717.1085;817.8743;918.6253;1019.36;1120.084;1220.799;1321.51;1422.22;1522.93;1623.639;1724.337;1824.924;1926.177;2026.763]  Table=[400;500;600;700;800;900;1000;1100;1200;1300;1400;1500;1600;1700;1800;1900;2000]  InternalRulePriority=Speed  RndMeth=Simplest
  Out1 : Outport
  wires:
  In1/1 -> LUT 0.87RR/1
  LUT 0.87RR/1 -> Out1/1

== system LUT_liver_pancreas_25/If Action Subsystem6/If Action Subsystem3/If Action Subsystem8/If Action Subsystem8 ==
  In1 : Inport
  Action Port : ActionPort  ActionPortLabel=elseif(u1 >= 0.875)
  LUT 0.88RR : Lookup_n-D  NumberOfTableDimensions=1  BreakpointsForDimension1=[405.0795;515.6172;615.9496;716.5762;817.2147;917.8359;1018.44;1119.03;1219.612;1320.188;1420.762;1521.334;1621.905;1722.466;1822.953;1924.179;2024.472]  Table=[400;500;600;700;800;900;1000;1100;1200;1300;1400;1500;1600;1700;1800;1900;2000]  InternalRulePriority=Speed  RndMeth=Simplest
  Out1 : Outport
  wires:
  In1/1 -> LUT 0.88RR/1
  LUT 0.88RR/1 -> Out1/1

== system LUT_liver_pancreas_25/If Action Subsystem6/If Action Subsystem3/If Action Subsystem8/If Action Subsystem9 ==
  In1 : Inport
  Action Port : ActionPort  ActionPortLabel=if(u1 >= 0.885)
  LUT 0.89RR : Lookup_n-D  NumberOfTableDimensions=1  BreakpointsForDimension1=[404.919;515.3366;615.5562;716.063;816.5779;917.0732;1017.55;1118.011;1218.463;1318.908;1419.349;1519.789;1620.226;1720.654;1821.029;1922.578;2022.259]  Table=[400;500;600;700;800;900;1000;1100;1200;1300;1400;1500;1600;1700;1800;1900;2000]  InternalRulePriority=Speed  RndMeth=Simplest
  Out1 : Outport
  wires:
  In1/1 -> LUT 0.89RR/1
  LUT 0.89RR/1 -> Out1/1

== system LUT_liver_pancreas_25/If Action Subsystem6/If Action Subsystem3/If Action Subsystem9/If Action Subsystem1 ==
  In1 : Inport
  Action Port : ActionPort  ActionPortLabel=elseif( u1 >= 0.915)
  LUT 0.92RR : Lookup_n-D  NumberOfTableDimensions=1  BreakpointsForDimension1=[404.4711;514.5547;614.4583;714.6274;814.7928;914.9313;1015.046;1115.142;1215.225;1315.298;1415.365;1515.427;1615.484;1715.534;1815.559;1915.336;2016.081]  Table=[400;500;600;700;800;900;1000;1100;1200;1300;1400;1500;1600;1700;1800;1900;2000]  InternalRulePriority=Speed  RndMeth=Simplest
  Out1 : Outport
  wires:
  In1/1 -> LUT 0.92RR/1
  LUT 0.92RR/1 -> Out1/1

== system LUT_liver_pancreas_25/If Action Subsystem6/If Action Subsystem3/If Action Subsystem9/If Action Subsystem10 ==
  In1 : Inport
  Action Port : ActionPort  ActionPortLabel=elseif( u1 >= 0.905)
  LUT 0.91RR : Lookup_n-D  NumberOfTableDimensions=1  BreakpointsForDimension1=[404.6151;514.8059;614.8113;715.0896;815.3681;915.6222;1015.854;1116.069;1216.271;1316.465;1416.653;1516.837;1617.018;1717.19;1817.331;1916.961;2018.061]  Table=[400;500;600;700;800;900;1000;1100;1200;1300;1400;1500;1600;1700;1800;1900;2000]  InternalRulePriority=Speed  RndMeth=Simplest
  Out1 : Outport
  wires:
  In1/1 -> LUT 0.91RR/1
  LUT 0.91RR/1 -> Out1/1

== system LUT_liver_pancreas_25/If Action Subsystem6/If Action Subsystem3/If Action Subsystem9/If Action Subsystem2 ==
  In1 : Inport
  Action Port : ActionPort  ActionPortLabel=else
  LUT 0.90RR : Lookup_n-D  NumberOfTableDimensions=1  BreakpointsForDimension1=[404.7643;515.0663;615.177;715.5678;815.9628;916.3358;1016.688;1117.025;1217.35;1317.668;1417.981;1518.291;1618.597;1718.896;1819.154;1923.465;2020.122]  Table=[400;500;600;700;800;900;1000;1100;1200;1300;1400;1500;1600;1700;1800;1900;2000]  InternalRulePriority=Speed  RndMeth=Simplest
  Out1 : Outport
  wires:
  In1/1 -> LUT 0.90RR/1
  LUT 0.90RR/1 -> Out1/1

== system LUT_liver_pancreas_25/If Action Subsystem6/If Action Subsystem3/If Action Subsystem9/If Action Subsystem3 ==
  In1 : Inport
  Action Port : ActionPort  ActionPortLabel=elseif( u1 >= 0.925)
  LUT 0.93RR : Lookup_n-D  NumberOfTableDimensions=1  BreakpointsForDimension1=[404.3319;514.3123;614.1172;714.1804;814.2358;914.2619;1014.262;1114.243;1214.209;1314.165;1414.113;1514.057;1613.995;1713.925;1813.834;1913.596;2014.202]  Table=[400;500;600;700;800;900;1000;1100;1200;1300;1400;1500;1600;1700;1800;1900;2000]  InternalRulePriority=Speed  RndMeth=Simplest
  Out1 : Outport
  wires:
  In1/1 -> LUT 0.93RR/1
  LUT 0.93RR/1 -> Out1/1

== system LUT_liver_pancreas_25/If Action Subsystem6/If Action Subsystem3/If Action Subsystem9/If Action Subsystem4 ==
  In1 : Inport
  Action Port : ActionPort  ActionPortLabel=elseif( u1 >= 0.935)
  LUT 0.94RR : Lookup_n-D  NumberOfTableDimensions=1  BreakpointsForDimension1=[404.1974;514.0782;613.7875;713.7478;813.6963;913.6128;1013.502;1113.37;1213.223;1313.064;1412.898;1512.725;1612.547;1712.361;1812.157;1911.855;2012.487]  Table=[400;500;600;700;800;900;1000;1100;1200;1300;1400;1500;1600;1700;1800;1900;2000]  InternalRulePriority=Speed  RndMeth=Simplest
  Out1 : Outport
  wires:
  In1/1 -> LUT 0.94RR/1
  LUT 0.94RR/1 -> Out1/1

== system LUT_liver_pancreas_25/If Action Subsystem6/If Action Subsystem3/If Action Subsystem9/If Action Subsystem5 ==
  In1 : Inport
  Action Port : ActionPort  ActionPortLabel=elseif( u1 >= 0.955)
  LUT 0.96RR : Lookup_n-D  NumberOfTableDimensions=1  BreakpointsForDimension1=[403.9412;513.6329;613.1599;712.923;812.6661;912.3722;1012.047;1111.699;1211.333;1310.954;1410.566;1510.171;1609.769;1709.359;1808.935;1908.458;2012.979]  Table=[400;500;600;700;800;900;1000;1100;1200;1300;1400;1500;1600;1700;1800;1900;2000]  InternalRulePriority=Speed  RndMeth=Simplest
  Out1 : Outport
  wires:
  In1/1 -> LUT 0.96RR/1
  LUT 0.96RR/1 -> Out1/1

== system LUT_liver_pancreas_25/If Action Subsystem6/If Action Subsystem3/If Action Subsystem9/If Action Subsystem6 ==
  In1 : Inport
  Action Port : ActionPort  ActionPortLabel=elseif( u1 >= 0.945)
  LUT 0.95RR : Lookup_n-D  NumberOfTableDimensions=1  BreakpointsForDimension1=[404.0672;513.8518;613.4686;713.3289;813.1733;912.9832;1012.764;1112.522;1212.265;1311.995;1411.716;1511.43;1611.139;1710.84;1810.525;1910.139;2011.266]  Table=[400;500;600;700;800;900;1000;1100;1200;1300;1400;1500;1600;1700;1800;1900;2000]  InternalRulePriority=Speed  RndMeth=Simplest
  Out1 : Outport
  wires:
  In1/1 -> LUT 0.95RR/1
  LUT 0.95RR/1 -> Out1/1

== system LUT_liver_pancreas_25/If Action Subsystem6/If Action Subsystem3/If Action Subsystem9/If Action Subsystem7 ==
  In1 : Inport
  Action Port : ActionPort  ActionPortLabel=elseif( u1 >= 0.965)
  LUT 0.97RR : Lookup_n-D  NumberOfTableDimensions=1  BreakpointsForDimension1=[403.8191;513.421;612.8609;712.5295;812.1739;911.7787;1011.351;1110.898;1210.427;1309.942;1409.448;1508.945;1608.435;1707.918;1807.387;1906.815;2005.674]  Table=[400;500;600;700;800;900;1000;1100;1200;1300;1400;1500;1600;1700;1800;1900;2000]  InternalRulePriority=Speed  RndMeth=Simplest
  Out1 : Outport
  wires:
  In1/1 -> LUT 0.97RR/1
  LUT 0.97RR/1 -> Out1/1

== system LUT_liver_pancreas_25/If Action Subsystem6/If Action Subsystem3/If Action Subsystem9/If Action Subsystem8 ==
  In1 : Inport
  Action Port : ActionPort  ActionPortLabel=elseif(u1 >= 0.975)
  LUT 0.98RR : Lookup_n-D  NumberOfTableDimensions=1  BreakpointsForDimension1=[403.7006;513.2158;612.5711;712.1478;811.6961;911.2022;1010.674;1110.119;1209.546;1308.957;1408.358;1507.751;1607.136;1706.513;1805.879;1905.21;2004.261]  Table=[400;500;600;700;800;900;1000;1100;1200;1300;1400;1500;1600;1700;1800;1900;2000]  InternalRulePriority=Speed  RndMeth=Simplest
  Out1 : Outport
  wires:
  In1/1 -> LUT 0.98RR/1
  LUT 0.98RR/1 -> Out1/1

== system LUT_liver_pancreas_25/If Action Subsystem6/If Action Subsystem3/If Action Subsystem9/If Action Subsystem9 ==
  In1 : Inport
  Action Port : ActionPort  ActionPortLabel=if(u1 >= 0.985)
  LUT 0.99RR : Lookup_n-D  NumberOfTableDimensions=1  BreakpointsForDimension1=[403.5857;513.0169;612.2901;711.7773;811.232;910.6418;1010.015;1109.361;1208.687;1307.998;1407.298;1506.588;1605.87;1705.145;1804.408;1903.644;2002.71]  Table=[400;500;600;700;800;900;1000;1100;1200;1300;1400;1500;1600;1700;1800;1900;2000]  InternalRulePriority=Speed  RndMeth=Simplest
  Out1 : Outport
  wires:
  In1/1 -> LUT 0.99RR/1
  LUT 0.99RR/1 -> Out1/1
